simulink model "vexarmcortex_BEST_SimBot_Autonomous_Chart"  (R2019a)
settings: Solver=FixedStepAuto  StartTime=0.0  StopTime=inf  RelTol=1e-3  EnableMultiTasking=on
libraries: vexarmcortexlib x13, vexcommonlib x2, simulink x1
settings Model: Creator=josea  LastModifiedBy=josea
settings DataIOCC: LimitDataPoints=on  SignalLoggingSaveFormat=ModelDataLogs  ReturnWorkspaceOutputs=off
settings OptimizationCC: ExpressionDepthLimit=2147483647  LifeSpan=Inf  MaxStackSize=64
settings DebuggingCC: UnderspecifiedInitializationDetection=Classic  MergeDetectMultiDrivingBlocksExec=none  InheritedTsInSrcMsg=none  FcnCallInpInsideContextMsg=warning  UnconnectedInputMsg=none  UnconnectedOutputMsg=none  StateNameClashWarn=warning  SFUnexpectedBacktrackingDiag=warning  SFNoUnconditionalDefaultTransitionDiag=warning  SFExecutionAtInitializationDiag=none  ArithmeticOperatorsInVariantConditions=warning
settings HardwareCC: ProdBitPerPointer=32  ProdBitPerSizeT=32  ProdBitPerPtrDiffT=32  ProdLargestAtomicInteger=Long  ProdLargestAtomicFloat=Double  ProdIntDivRoundTo=Undefined  ProdWordSize=32  ProdHWDeviceType=ARM Compatible->ARM Cortex
settings ModelReferenceCC: PropagateSignalLabelsOutOfModel=off
settings SFSimCC: MATLABDynamicMemAlloc=off
settings RTWCC: SystemTargetFile=ert.tlc  HardwareBoard=ARM Cortex-based VEX Microcontroller  TemplateMakefile=ert_default_tmf  Toolchain=GNU Tools for VEX ARM Cortex
settings CodeAppCC: IgnoreCustomStorageClasses=off  CustomSymbolStrType=$N$R$M  StateflowObjectComments=on  InternalIdentifier=Classic
settings ERTTargetCC: CodeReplacementLibrary=GCC ARM Cortex-M3  MultiwordLength=2048  ConvertIfToSwitch=off  SuppressUnreachableDefaultCases=off

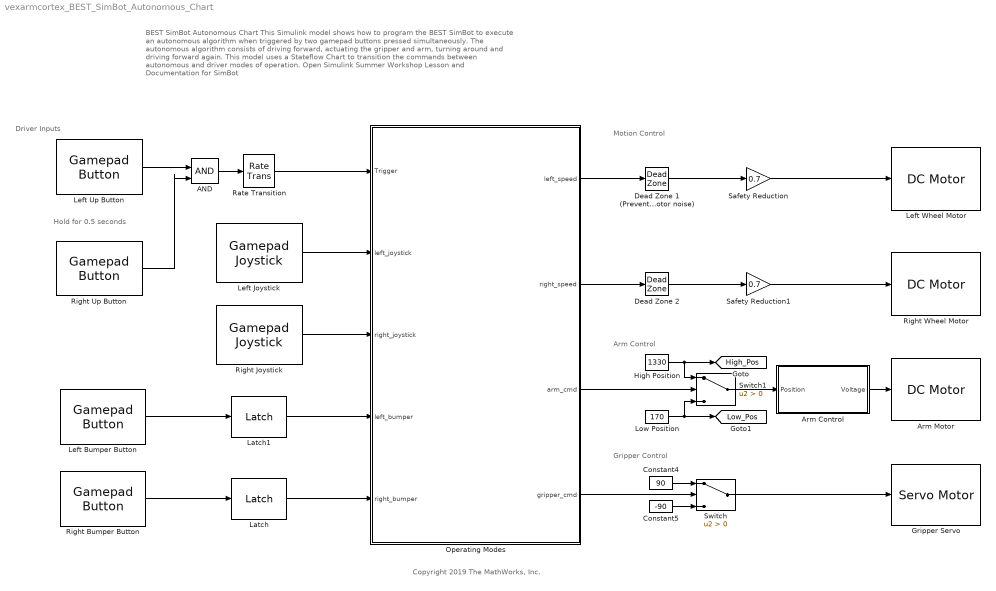
== system vexarmcortex_BEST_SimBot_Autonomous_Chart ==
  note: Hold for 0.5 seconds
  note: Driver Inputs
  note: Copyright 2019 The MathWorks, Inc.
  note: BEST SimBot Autonomous Chart
      | This Simulink model shows how to program the BEST SimBot to execute an autonomous algorithm
      | when triggered by two gamepad buttons pressed simultaneously. The autonomous algorithm consists of driving forward,
      | actuating the gripper and arm, turning around and driving forward again. This model uses a Stateflow Chart to transition
      | the commands between autonomous and driver modes of operation.
      | Open Simulink Summer Workshop Lesson and Documentation for SimBot
  note: Gripper Control
  note: Motion Control
  note: Arm Control
  AND : Logic  IconShape=distinctive  AllPortsSameDT=off  OutDataTypeStr=boolean
  Arm Control : Subsystem
  Arm Motor : vexarmcortexlib/Actuators/DC Motor  motor=4  scaleFactor=1/13.5  SimulationOut=off
      settings: SourceProductName=Simulink Coder Support Package for ARM Cortex-based VEX Microcontroller  SourceProductBaseCode=EC_VEX_MICRO
  Constant4 : Constant  Value=90
  Constant5 : Constant  Value=-90
  Dead Zone 1 (Prevents motor noise) : DeadZone  LowerValue=-30  UpperValue=30  SaturateOnIntegerOverflow=on
  Dead Zone 2 : DeadZone  LowerValue=-30  UpperValue=30  SaturateOnIntegerOverflow=on
  Gripper Servo : vexarmcortexlib/Actuators/Servo Motor  motor=2  scaleFactor=60/127  SimulationOut=off
      settings: SourceProductName=Simulink Coder Support Package for ARM Cortex-based VEX Microcontroller  SourceProductBaseCode=EC_VEX_MICRO
  High Position : Constant  Value=1330
  Latch : vexcommonlib/Latch  output0=off  BlockPlatform=vexarmcortex
      settings: SourceProductName=Simulink Coder Support Package for ARM Cortex-based VEX Microcontroller  SourceProductBaseCode=EC_VEX_MICRO
  Latch1 : vexcommonlib/Latch  output0=off  BlockPlatform=vexarmcortex
      settings: SourceProductName=Simulink Coder Support Package for ARM Cortex-based VEX Microcontroller  SourceProductBaseCode=EC_VEX_MICRO
  Left Bumper Button : vexarmcortexlib/Gamepad/Gamepad Button  joystick=1  chan=6  button56=Up  button78=Down  SimulationIn=off  SampleTime=0.02
      settings: SourceProductName=Simulink Coder Support Package for ARM Cortex-based VEX Microcontroller  SourceProductBaseCode=EC_VEX_MICRO
  Left Joystick : vexarmcortexlib/Gamepad/Gamepad Joystick  joystick=1  chan=3  SimulationIn=off  SampleTime=0.02
      settings: SourceProductName=Simulink Coder Support Package for ARM Cortex-based VEX Microcontroller  SourceProductBaseCode=EC_VEX_MICRO
  Left Up Button : vexarmcortexlib/Gamepad/Gamepad Button  joystick=1  chan=7  button56=Down  button78=Up  SimulationIn=off  SampleTime=0.5
      settings: SourceProductName=Simulink Coder Support Package for ARM Cortex-based VEX Microcontroller  SourceProductBaseCode=EC_VEX_MICRO
  Left Wheel Motor : vexarmcortexlib/Actuators/DC Motor  motor=5  scaleFactor=1/13.5  SimulationOut=off
      settings: SourceProductName=Simulink Coder Support Package for ARM Cortex-based VEX Microcontroller  SourceProductBaseCode=EC_VEX_MICRO
  Low Position : Constant  Value=170
  Operating Modes : Stateflow chart  TreatAsAtomicUnit=on
  Rate Transition : RateTransition
  Right Bumper Button : vexarmcortexlib/Gamepad/Gamepad Button  joystick=1  chan=5  button56=Up  button78=Down  SimulationIn=off  SampleTime=0.02
      settings: SourceProductName=Simulink Coder Support Package for ARM Cortex-based VEX Microcontroller  SourceProductBaseCode=EC_VEX_MICRO
  Right Joystick : vexarmcortexlib/Gamepad/Gamepad Joystick  joystick=1  chan=2  SimulationIn=off  SampleTime=0.02
      settings: SourceProductName=Simulink Coder Support Package for ARM Cortex-based VEX Microcontroller  SourceProductBaseCode=EC_VEX_MICRO
  Right Up Button : vexarmcortexlib/Gamepad/Gamepad Button  joystick=1  chan=8  button56=Down  button78=Up  SimulationIn=off  SampleTime=0.5
      settings: SourceProductName=Simulink Coder Support Package for ARM Cortex-based VEX Microcontroller  SourceProductBaseCode=EC_VEX_MICRO
  Right Wheel Motor : vexarmcortexlib/Actuators/DC Motor  motor=3  scaleFactor=1/13.5  SimulationOut=off
      settings: SourceProductName=Simulink Coder Support Package for ARM Cortex-based VEX Microcontroller  SourceProductBaseCode=EC_VEX_MICRO
  Safety Reduction : Gain  Gain=0.7
  Safety Reduction1 : Gain  Gain=0.7
  Switch : Switch  Criteria=u2 > Threshold
  Switch1 : Switch  Criteria=u2 > Threshold
  tag scope: High_Pos=global, Low_Pos=global
  wires:
  Right Up Button/1 -> AND/2
  Left Up Button/1 -> AND/1
  Switch1/1 -> Arm Control/1(Position)
  Arm Control/1(Voltage) -> Arm Motor/1
  Constant4/1 -> Switch/1
  Low Position/1 -> [Low_Pos], Switch1/3
  Dead Zone 2/1 -> Safety Reduction1/1
  Constant5/1 -> Switch/3
  Switch/1 -> Gripper Servo/1
  High Position/1 -> [High_Pos], Switch1/1
  Dead Zone 1 (Prevents motor noise)/1 -> Safety Reduction/1
  Safety Reduction/1 -> Left Wheel Motor/1
  Safety Reduction1/1 -> Right Wheel Motor/1
  AND/1 -> Rate Transition/1
  Left Joystick/1 -> Operating Modes/2(left_joystick)
  Right Joystick/1 -> Operating Modes/3(right_joystick)
  Left Bumper Button/1 -> Latch1/1
  Right Bumper Button/1 -> Latch/1
  Operating Modes/1(left_speed) -> Dead Zone 1 (Prevents motor noise)/1
  Operating Modes/2(right_speed) -> Dead Zone 2/1
  Rate Transition/1 -> Operating Modes/1(Trigger)
  Latch1/1 -> Operating Modes/4(left_bumper)
  Latch/1 -> Operating Modes/5(right_bumper)
  Operating Modes/3(arm_cmd) -> Switch1/2
  Operating Modes/4(gripper_cmd) -> Switch/2

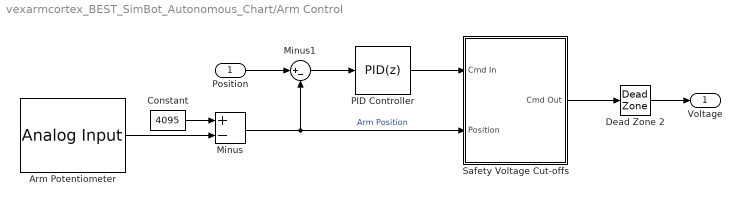
== system vexarmcortex_BEST_SimBot_Autonomous_Chart/Arm Control ==
  Position : Inport
  Arm Potentiometer : vexarmcortexlib/Sensors/Analog Input  inChan=1  SimulationIn=off  SampleTime=0.02
      settings: SourceProductName=Simulink Coder Support Package for ARM Cortex-based VEX Microcontroller  SourceProductBaseCode=EC_VEX_MICRO
  Constant : Constant  Value=4095
  Dead Zone 2 : DeadZone  LowerValue=-30  UpperValue=30  SaturateOnIntegerOverflow=on
  Minus : Sum  Inputs=+-
  Minus1 : Sum  Inputs=|+-
  PID Controller : simulink/Continuous/PID Controller  Controller=PID  Form=Parallel  TimeDomain=Discrete-time  SampleTime=-1  IntegratorMethod=Forward Euler  FilterMethod=Forward Euler  ControllerParametersSource=internal  P=1  I=0  D=0  UseFilter=on  N=100  TunerSelectOption=Transfer Function Based (PID Tuner App)  InitialConditionSource=internal  InitialConditionForIntegrator=0  InitialConditionForFilter=0  DifferentiatorICPrevScaledInput=0  ExternalReset=none  TrackingMode=off  Kt=1  LimitOutput=on  UpperSaturationLimit=127  LowerSaturationLimit=-127  LinearizeAsGain=on  AntiWindupMode=none  Kb=1  POutMin=[]  POutMax=[]  IOutMin=[]  IOutMax=[]  DOutMin=[]  DOutMax=[]  NOutMin=[]  NOutMax=[]  SumOutMin=[]  SumOutMax=[]  SaturationOutMin=[]  SaturationOutMax=[]  PParamMin=[]  PParamMax=[]  IParamMin=[]  IParamMax=[]  DParamMin=[]  DParamMax=[]  NParamMin=[]  NParamMax=[]  KbParamMin=[]  KbParamMax=[]  KtParamMin=[]  KtParamMax=[]  KbOutMin=[]  KbOutMax=[]  KtOutMin=[]  KtOutMax=[]  IntegratorOutMin=[]  IntegratorOutMax=[]  FilterOutMin=[]  FilterOutMax=[]  SumI1OutMin=[]  SumI1OutMax=[]  SumI2OutMin=[]  SumI2OutMax=[]  SumI3OutMin=[]  SumI3OutMax=[]  SumI4OutMin=[]  SumI4OutMax=[]  SumDOutMin=[]  SumDOutMax=[]  DifferentiatorOutMin=[]  DifferentiatorOutMax=[]  FilterDiffOutCoefMin=[]  FilterDiffOutCoefMax=[]  ReciprocalOutMin=[]  ReciprocalOutMax=[]  SumDenOutMin=[]  SumDenOutMax=[]  SumNumOutMin=[]  SumNumOutMax=[]  DivideOutMin=[]  DivideOutMax=[]  IntegratorContinuousStateAttributes=''  IntegratorStateMustResolveToSignalObject=off  IntegratorRTWStateStorageClass=Auto  FilterContinuousStateAttributes=''  FilterStateMustResolveToSignalObject=off  FilterRTWStateStorageClass=Auto  ParallelPVariant=InternalParameters  IdealPVariant=Disabled  IVariant=InternalParameters  DVariant=InternalParameters  IntegratorVariant=Discrete  SatVariant=Enabled  AWVariant=Passthrough  PCopyVariant=Disabled  TRVariant=Disabled  FdbkBlocksVariant=Forward  IdealPFdbkVariant=Disabled  SatFdbkVariant=Disabled  DerivativeFilterVariant=ForwardEulerFilter  NVariant=InternalParameters  NCopyVariant=Disabled  FilterICVariant=InternalICsFilter  IntegratorICVariant=InternalICs  ExternalResetVariant=Disabled  TRSumVariant=Passthrough  SumFdbkVariant=Disabled  SumVariant=Sum_PID
  Safety Voltage Cut-offs : Subsystem
  Voltage : Outport
  wires:
  Dead Zone 2/1 -> Voltage/1
  Safety Voltage Cut-offs/1(Cmd Out) -> Dead Zone 2/1
  PID Controller/1 -> Safety Voltage Cut-offs/1(Cmd In)
  Position/1 -> Minus1/1
  Arm Potentiometer/1 -> Minus/2
  Constant/1 -> Minus/1
  Minus1/1 -> PID Controller/1
  Minus/1 -> Safety Voltage Cut-offs/2(Position), Minus1/2  "Arm Position"

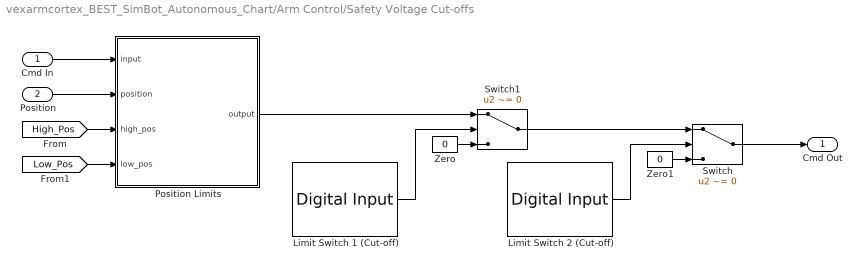
== system vexarmcortex_BEST_SimBot_Autonomous_Chart/Arm Control/Safety Voltage Cut-offs ==
  Cmd In : Inport
  Position : Inport  Port=2
  Limit Switch 1 (Cut-off) : vexarmcortexlib/Sensors/Digital Input  inChan=1  SimulationIn=off  SampleTime=0.02
      settings: SourceProductName=Simulink Coder Support Package for ARM Cortex-based VEX Microcontroller  SourceProductBaseCode=EC_VEX_MICRO
  Limit Switch 2 (Cut-off) : vexarmcortexlib/Sensors/Digital Input  inChan=2  SimulationIn=off  SampleTime=0.02
      settings: SourceProductName=Simulink Coder Support Package for ARM Cortex-based VEX Microcontroller  SourceProductBaseCode=EC_VEX_MICRO
  Position Limits : MATLAB Function  TreatAsAtomicUnit=on
  Switch : Switch  Criteria=u2 ~= 0
  Switch1 : Switch  Criteria=u2 ~= 0
  Zero : Constant  Value=0  OutDataTypeStr=Inherit: Inherit via back propagation
  Zero1 : Constant  Value=0  OutDataTypeStr=Inherit: Inherit via back propagation
  Cmd Out : Outport
  wires:
  [Low_Pos] -> Position Limits/4(low_pos)
  [High_Pos] -> Position Limits/3(high_pos)
  Switch/1 -> Cmd Out/1
  Zero/1 -> Switch1/3
  Cmd In/1 -> Position Limits/1(input)
  Position Limits/1(output) -> Switch1/1
  Limit Switch 2 (Cut-off)/1 -> Switch/2
  Zero1/1 -> Switch/3
  Switch1/1 -> Switch/1
  Limit Switch 1 (Cut-off)/1 -> Switch1/2
  Position/1 -> Position Limits/2(position)

== matlab function vexarmcortex_BEST_SimBot_Autonomous_Chart/Arm Control/Safety Voltage Cut-offs/Position Limits ==
  data: input input; output output; position input; high_pos input; low_pos input
function output = armLimits(input, position, high_pos, low_pos)

if input >0 && position < high_pos+50 %Highest safe arm position
    output=input;
elseif input <0 && position > low_pos-50 %Lowest safe arm position
    output=input;
else
    output=0;
end

end

== stateflow chart vexarmcortex_BEST_SimBot_Autonomous_Chart/Operating Modes ==
  state DriverControl
    left_speed = left_joystick;
    right_speed = right_joystick;
    arm_cmd = left_bumper;
    gripper_cmd = right_bumper;
  state AutonomousMode
    state MoveForward
      en:
      right_speed = 90;
      left_speed = 90;
    state TurnAround
      en:
      right_speed = 90;
      left_speed = -90;
    state MoveBackward
      en:
      right_speed = 90;
      left_speed = 90;
    state Stop
      en:
      right_speed = 0;
      left_speed = 0;
      Done = true;
    (default) -> MoveForward : {Done = false;
        | gripper_cmd = 0;
        | arm_cmd=0;}
    MoveForward -> TurnAround : after(4,sec)
    TurnAround -> MoveBackward : after(6,sec)
    MoveBackward -> Stop : after(4,sec)
  (default) -> DriverControl
  DriverControl -> AutonomousMode : [Trigger]
  AutonomousMode -> DriverControl : [Trigger || Done]
  data: Trigger input; left_joystick input; right_joystick input; left_bumper input; right_bumper input; left_speed output; right_speed output; arm_cmd output; gripper_cmd output; Done local boolean
